simulink model "stm32f207_template_app"  (R2023b)
settings: Solver=FixedStepDiscrete  StartTime=0.0  StopTime=10.0  FixedStep=0.01  RelTol=1e-3
model workspace (MAT data in the model file):
  BlueSwitch = Simulink.Parameter
  BlueSwitch.Value = 1
  BlueSwitch.DataType = 'boolean'
  BlueSwitch.Complexity = 'real'
  BlueSwitch.Dimensions = [1 1]
  GreenSwitch = Simulink.Parameter
  GreenSwitch.Value = 0
  GreenSwitch.DataType = 'boolean'
  GreenSwitch.Complexity = 'real'
  GreenSwitch.Dimensions = [1 1]
  RedSwitch = Simulink.Parameter
  RedSwitch.Value = 1
  RedSwitch.DataType = 'boolean'
  RedSwitch.Complexity = 'real'
  RedSwitch.Dimensions = [1 1]
libraries: canmsglib x5, can_control x5, led_control x3, simulink x2
settings Model: Creator=Professional  LastModifiedBy=Olga
settings SolverCC: AutoInsertRateTranBlk=on
settings OptimizationCC: DefaultParameterBehavior=Inlined  UseDivisionForNetSlopeComputation=on  GainParamInheritBuiltInType=on  UseFloatMulNetSlope=on  DefaultUnderspecifiedDataType=single  UseSpecifiedMinMax=on  InlineInvariantSignals=on  BitwiseOrLogicalOp=Bitwise operator  PassReuseOutputArgsAs=Individual arguments  ZeroExternalMemoryAtStartup=off  ZeroInternalMemoryAtStartup=off  NoFixptDivByZeroProtection=on  EfficientFloat2IntCast=on  LifeSpan=inf  OptimizeBlockOrder=speed  DifferentSizesBufferReuse=on  EfficientTunableParamExpr=on
settings DebuggingCC: SignalInfNanChecking=warning  WriteAfterWriteMsg=EnableAllAsError  InheritedTsInSrcMsg=none  MultiTaskDSMMsg=none  IntegerOverflowMsg=error  ParameterPrecisionLossMsg=none  ParameterTunabilityLossMsg=error  UniqueDataStoreMsg=error  AssertControl=DisableAll  ModelReferenceSymbolNameMessage=none  NonBusSignalsTreatedAsBus=error  SFInvalidInputDataAccessInChartInitDiag=error  SFTransitionOutsideNaturalParentDiag=error  SFUnreachableExecutionPathDiag=error  SFUndirectedBroadcastEventsDiag=error  IntegerSaturationMsg=error
settings HardwareCC: ProdBitPerPointer=32  ProdBitPerSizeT=32  ProdBitPerPtrDiffT=32  ProdLargestAtomicInteger=Long  ProdLargestAtomicFloat=Double  ProdWordSize=32  ProdHWDeviceType=ARM Compatible->ARM Cortex-M
settings ModelReferenceCC: ModelReferenceNumInstancesAllowed=Single
settings SFSimCC: CompileTimeRecursionLimit=0  EnableRuntimeRecursion=off  MATLABDynamicMemAlloc=off
settings RTWCC: Description=Embedded Coder  SystemTargetFile=ert.tlc  GenCodeOnly=on  PackageGeneratedCodeAndArtifacts=on  PackageName=simulink_app  TemplateMakefile=ert_default_tmf  GenerateReport=on  CustomHeaderCode="#include \"rtmodel.h\""  IncludeHyperlinkInReport=on  LaunchReport=on  GenerateTraceInfo=on  GenerateTraceReport=on  GenerateTraceReportSl=on  GenerateTraceReportSf=on  GenerateTraceReportEml=on
settings CodeAppCC: ForceParamTrailComments=on  IgnoreCustomStorageClasses=off  OperatorAnnotations=on  SimulinkDataObjDesc=on  SFDataObjDesc=on  MATLABFcnDesc=on  InsertBlockDesc=on  StateflowObjectComments=on  MATLABSourceComments=on  EnableCustomComments=on  ReqsInCode=on
settings ERTTargetCC: TargetLangStandard=C99 (ISO)  UtilityFuncGeneration=Shared location  CombineSignalStateStructs=on  SuppressErrorStatus=on  SupportNonFinite=off  SupportComplex=off  ParenthesesLevel=Standards  CastingMode=Standards  ERTHeaderFileRootName=$Usimulink_app$E  ERTSourceFileRootName=$Usimulink_app$E  InlinedParameterPlacement=NonHierarchical  ERTCustomFileTemplate=example_file_process.tlc  SuppressUnreachableDefaultCases=off  EnableSignedLeftShifts=off  EnableSignedRightShifts=off

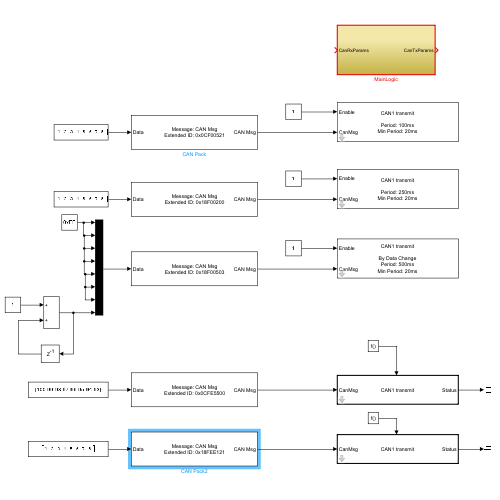
[thumbnail: Simulink's stored preview of the top-level diagram]
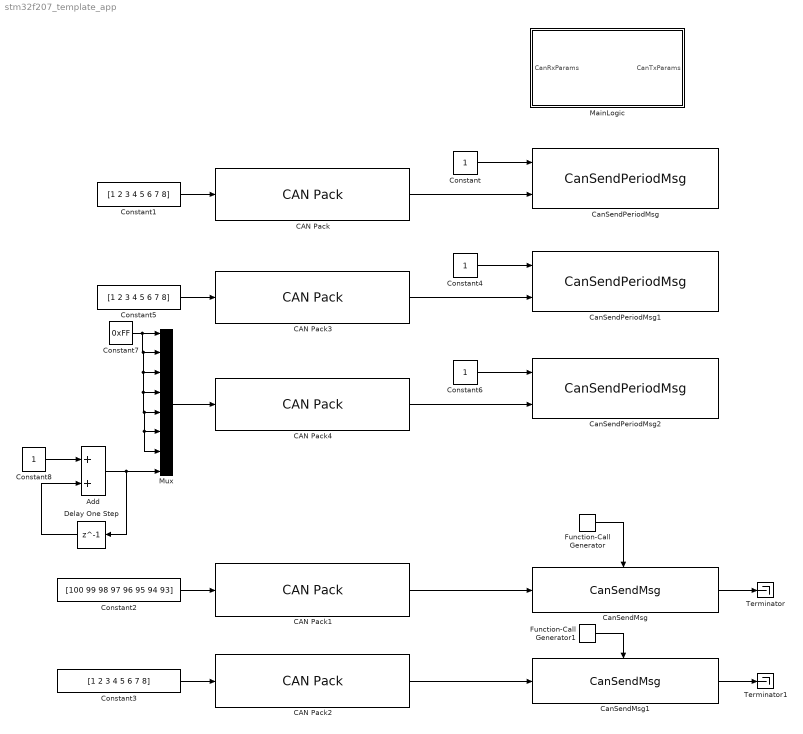
== system stm32f207_template_app ==
  Add : Sum  AccumDataTypeStr=uint8  RndMeth=Simplest
  CAN Pack : canmsglib/CAN Pack  MsgList=(none)  MsgName=CAN Msg  MsgIDType=Extended (29-bit identifier)  MsgIdentifier=0x0CF00521  MsgLength=8  Remote=off  ApplyMinMax=off  BusOutput=on  SignalInfo={}
      settings: LibrarySourceBlock=embeddedtargetslib/Host Communication/CAN Pack  DataFormat=raw data
  CAN Pack1 : canmsglib/CAN Pack  MsgList=(none)  MsgName=CAN Msg  MsgIDType=Extended (29-bit identifier)  MsgIdentifier=0x0CFE5500  MsgLength=8  Remote=off  ApplyMinMax=off  BusOutput=on  SignalInfo={}
      settings: LibrarySourceBlock=embeddedtargetslib/Host Communication/CAN Pack  DataFormat=raw data
  CAN Pack2 : canmsglib/CAN Pack  MsgList=(none)  MsgName=CAN Msg  MsgIDType=Extended (29-bit identifier)  MsgIdentifier=0x18FEE121  MsgLength=8  Remote=off  ApplyMinMax=off  BusOutput=on  SignalInfo={}
      settings: LibrarySourceBlock=embeddedtargetslib/Host Communication/CAN Pack  DataFormat=raw data
  CAN Pack3 : canmsglib/CAN Pack  MsgList=(none)  MsgName=CAN Msg  MsgIDType=Extended (29-bit identifier)  MsgIdentifier=0x18F00200  MsgLength=8  Remote=off  ApplyMinMax=off  BusOutput=on  SignalInfo={}
      settings: LibrarySourceBlock=embeddedtargetslib/Host Communication/CAN Pack  DataFormat=raw data
  CAN Pack4 : canmsglib/CAN Pack  MsgList=(none)  MsgName=CAN Msg  MsgIDType=Extended (29-bit identifier)  MsgIdentifier=0x18F00503  MsgLength=8  Remote=off  ApplyMinMax=off  BusOutput=on  SignalInfo={}
      settings: LibrarySourceBlock=embeddedtargetslib/Host Communication/CAN Pack  DataFormat=raw data
  Constant : Constant  OutDataTypeStr=boolean
  Constant1 : Constant  Value=[1 2 3 4 5 6 7 8]  OutDataTypeStr=uint8
  Constant2 : Constant  Value=[100 99 98 97 96 95 94 93]  OutDataTypeStr=uint8
  Constant3 : Constant  Value=[1 2 3 4 5 6 7 8]  OutDataTypeStr=uint8
  Constant4 : Constant  OutDataTypeStr=boolean
  Constant5 : Constant  Value=[1 2 3 4 5 6 7 8]  OutDataTypeStr=uint8
  Constant6 : Constant  OutDataTypeStr=boolean
  Constant7 : Constant  Value=0xFF  OutDataTypeStr=uint8
  Constant8 : Constant  OutDataTypeStr=uint8
  Delay One Step : Delay  DelayLength=1  InitialCondition=0
  Function-Call Generator : simulink/Ports & Subsystems/Function-Call Generator  sample_time=1  numberOfIterations=1  DisallowWideOutput=off
  Function-Call Generator1 : simulink/Ports & Subsystems/Function-Call Generator  sample_time=0.5  numberOfIterations=1  DisallowWideOutput=off
  MainLogic : Subsystem  TreatAsAtomicUnit=on
      settings: RTWSystemCode=Inline
  Mux : Mux  Inputs=8
  Terminator : Terminator
  Terminator1 : Terminator
  СanSendMsg : can_control/СanSendMsg  can=CAN1
  СanSendMsg1 : can_control/СanSendMsg  can=CAN1
  СanSendPeriodMsg : can_control/СanSendPeriodMsg  by_period=on  by_dataChange=off  can=CAN1  period_time=0.1  sample_time=0.02
  СanSendPeriodMsg1 : can_control/СanSendPeriodMsg  by_period=on  by_dataChange=off  can=CAN1  period_time=0.25  sample_time=0.02
  СanSendPeriodMsg2 : can_control/СanSendPeriodMsg  by_period=on  by_dataChange=on  can=CAN1  period_time=0.5  sample_time=0.02
  wires:
  Constant/1 -> СanSendPeriodMsg/1
  CAN Pack/1 -> СanSendPeriodMsg/2
  Constant1/1 -> CAN Pack/1
  Constant2/1 -> CAN Pack1/1
  CAN Pack1/1 -> СanSendMsg/1
  CAN Pack2/1 -> СanSendMsg1/1
  Constant3/1 -> CAN Pack2/1
  СanSendMsg/1 -> Terminator/1
  СanSendMsg1/1 -> Terminator1/1
  Function-Call Generator/1 -> СanSendMsg/Trigger
  Function-Call Generator1/1 -> СanSendMsg1/Trigger
  Constant5/1 -> CAN Pack3/1
  CAN Pack3/1 -> СanSendPeriodMsg1/2
  Constant4/1 -> СanSendPeriodMsg1/1
  Constant6/1 -> СanSendPeriodMsg2/1
  CAN Pack4/1 -> СanSendPeriodMsg2/2
  Mux/1 -> CAN Pack4/1
  Constant7/1 -> Mux/7, Mux/6, Mux/5, Mux/4, Mux/3, Mux/2, Mux/1
  Add/1 -> Delay One Step/1, Mux/8
  Constant8/1 -> Add/1
  Delay One Step/1 -> Add/2

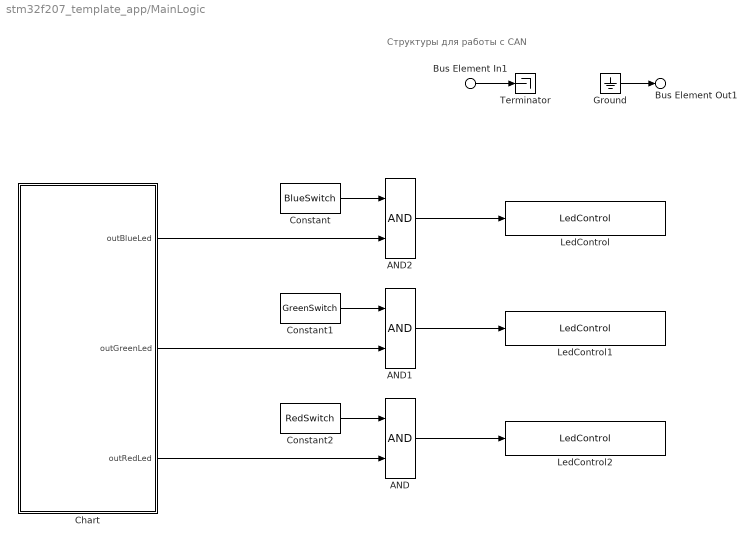
== system stm32f207_template_app/MainLogic ==
  note: Структуры для работы с CAN
  Bus Element In1 : Inport  PortName=CanRxParams
  AND : Logic  AllPortsSameDT=off  OutDataTypeStr=boolean
  AND1 : Logic  AllPortsSameDT=off  OutDataTypeStr=boolean
  AND2 : Logic  AllPortsSameDT=off  OutDataTypeStr=boolean
  Chart : Stateflow chart  TreatAsAtomicUnit=on
  Constant : Constant  Value=BlueSwitch
  Constant1 : Constant  Value=GreenSwitch
  Constant2 : Constant  Value=RedSwitch
  Ground : Ground
  LedControl : led_control/LedControl  Led=Blue
  LedControl1 : led_control/LedControl  Led=Green
  LedControl2 : led_control/LedControl  Led=Red
  Terminator : Terminator
  Bus Element Out1 : Outport  PortName=CanTxParams
  wires:
  Bus Element In1/1 -> Terminator/1
  Ground/1 -> Bus Element Out1/1
  Chart/3(outRedLed) -> AND/2
  Constant2/1 -> AND/1
  AND2/1 -> LedControl/1
  Constant/1 -> AND2/1
  Chart/1(outBlueLed) -> AND2/2
  Constant1/1 -> AND1/1
  Chart/2(outGreenLed) -> AND1/2
  AND1/1 -> LedControl1/1
  AND/1 -> LedControl2/1

== stateflow chart stm32f207_template_app/MainLogic/Chart ==
  state RED_LED [parallel]
    settings: executionOrder=1
    state OFF
      en:
      outRedLed = true;
    state ON
      en:
      outRedLed = false;
    (default) -> RED_LED.OFF
    RED_LED.OFF -> RED_LED.ON : after(100, msec)
    RED_LED.ON -> RED_LED.OFF : after(250, msec)
  state BLUE_LED [parallel]
    settings: executionOrder=2
    state OFF
      en:
      outBlueLed = true;
    state ON
      en:
      outBlueLed = false;
    (default) -> BLUE_LED.OFF
    BLUE_LED.OFF -> BLUE_LED.ON : after(500, msec)
    BLUE_LED.ON -> BLUE_LED.OFF : after(500, msec)
  state GREEN_LED [parallel]
    settings: executionOrder=3
    state OFF
      en:
      outGreenLed = true;
    state ON
      en:
      outGreenLed = false;
    (default) -> GREEN_LED.OFF
    GREEN_LED.OFF -> GREEN_LED.ON : after(1000, msec)
    GREEN_LED.ON -> GREEN_LED.OFF : after(1000, msec)
  data: outBlueLed output boolean; outGreenLed output boolean; outRedLed output boolean
